simulink model "Appl_DrRestMode_CtrlModel"  (R2018b)
settings: configuration reference "CodeConfig_10_ms" (kept outside this file)
undefined symbols (not defined in the file): D_ClickNapBackPosi, D_ClickNapLengthPosi, D_DRMEM_SPEED_5, D_SoftDistanceDrLegnth, FALSE, TRUE
libraries: DareLib x81, simulink x1
(part 2 of 2)

== system Appl_DrRestMode_CtrlModel/UpDataInputInfo/InputSignalProcess2/MotorFault ==
  CC4_Flag : Inport
  MotorFault_Flag : Stateflow chart  TreatAsAtomicUnit=on
  "MotroFault_Flag " : Outport
  wires:
  MotorFault_Flag/1(MotroFault_Flag) -> "MotroFault_Flag "/1
  CC4_Flag/1 -> MotorFault_Flag/1(CC4_Flag)

== system Appl_DrRestMode_CtrlModel/UpDataInputInfo/InputSignalProcess2/OPEN ==
  CC1_Flag : Inport
  DrRes_AnyoneRelayFaultSts : Inport  Port=2
  DrRes_MassageMode_FB : Inport  Port=3
  DrRes_IVI_NapMode_SwtichSet : Inport  Port=4
  Open_Flag : Stateflow chart  TreatAsAtomicUnit=on
  "Open_Flag " : Outport
  Open_Flag_Reason : Outport  Port=2
  wires:
  DrRes_MassageMode_FB/1 -> Open_Flag/1(DrRes_MassageMode_FB)
  CC1_Flag/1 -> Open_Flag/2(CC1_Flag)
  DrRes_AnyoneRelayFaultSts/1 -> Open_Flag/4(DrRes_AnyoneRelayFaultSts)
  Open_Flag/1(Open_Flag) -> "Open_Flag "/1
  Open_Flag/2(Open_Flag_Reason) -> Open_Flag_Reason/1
  DrRes_IVI_NapMode_SwtichSet/1 -> Open_Flag/3(DrRes_IVI_NapMode_SwtichSet)

== system Appl_DrRestMode_CtrlModel/UpDataInputInfo/InputSignalProcess2/STOP ==
  DrRes_VoltMode : Inport
  CC2_Flag : Inport  Port=2
  DrRes_VoltSatisfy : Inport  Port=3
  Stop_Flag : Stateflow chart  TreatAsAtomicUnit=on
  "Stop_Flag " : Outport
  Stop_Flag_Reason : Outport  Port=2
  wires:
  Stop_Flag/2(Stop_Flag_Reason) -> Stop_Flag_Reason/1
  DrRes_VoltMode/1 -> Stop_Flag/2(DrRes_VoltMode)
  CC2_Flag/1 -> Stop_Flag/1(CC2_Flag)
  Stop_Flag/1(Stop_Flag) -> "Stop_Flag "/1
  DrRes_VoltSatisfy/1 -> Stop_Flag/3(DrRes_VoltSatisfy)

== stateflow chart Appl_DrRestMode_CtrlModel/UpDataInputInfo/InputSignalProcess1/CC3/CC3_Flag ==
  state Init
    en:
    CC3_Flag = FALSE;
  state TRUE
    en:
    CC3_Flag = TRUE;
    CC3_Reason = FALSE;
  state FALSE
    en:
    CC3_Flag = FALSE;
  Init -> TRUE [order 4] : /* !PC2 ||!PC8 ||（!PC9 && !PC10 ）
      | 诊断F101中配置字：“座椅按摩功能”！= 0x01:Ture
      | ||系统电源不处于ON档
      | ||（收到发动机为ECMD_EngineStatus！=0x2=engine running；（仅当DID F1FA中配置字：“P20PHEV_100km & P20PHEV_50km”=0x00：False时适用）
      | && 收到整车运行状态为VCU_VehRunSta！= 0x1:HV ON /0x2:Ready；（仅当DID F1FA中配置字：“P20PHEV_100km / P20PHEV_50km”=0x01：Ture时适用）） */
      | [DrRes_SeatMassageCfg != TRUE...
      | || DrRes_PowerMode != enPowerModeSts.EN_ON ...
      | || (DrRes_EngineRunFlag == TRUE || DrRes_VehicleRunFlag == TRUE) ]
  (default) -> Init
  FALSE -> TRUE : /* !PC2 ||!PC8 ||（!PC9 && !PC10 ）
      | 诊断F101中配置字：“座椅按摩功能”！= 0x01:Ture
      | ||系统电源不处于ON档
      | ||（收到发动机为ECMD_EngineStatus！=0x2=engine running；（仅当DID F1FA中配置字：“P20PHEV_100km & P20PHEV_50km”=0x00：False时适用）
      | && 收到整车运行状态为VCU_VehRunSta！= 0x1:HV ON /0x2:Ready；（仅当DID F1FA中配置字：“P20PHEV_100km / P20PHEV_50km”=0x01：Ture时适用）） */
      | [DrRes_SeatMassageCfg != TRUE...
      | || DrRes_PowerMode != enPowerModeSts.EN_ON ...
      | || (DrRes_EngineRunFlag != TRUE && DrRes_VehicleRunFlag != TRUE) ]
  Init -> FALSE [order 1] : /*CC3未置位原因 ：DrRes_SeatMassageCfg 不满足条件 */
      | [DrRes_SeatMassageCfg == TRUE]
      | {CC3_Reason = 1}
  TRUE -> FALSE [order 1] : /*CC3未置位原因 ：DrRes_SeatMassageCfg 不满足条件 */
      | [DrRes_SeatMassageCfg == TRUE]
      | {CC3_Reason = 1}
  Init -> FALSE [order 2] : /*CC3未置位原因 ：DrRes_PowerMode 不满足条件*/
      | [DrRes_PowerMode == enPowerModeSts.EN_ON]
      | {CC3_Reason = 2}
  TRUE -> FALSE [order 2] : /*CC3未置位原因 ：DrRes_PowerMode 不满足条件*/
      | [DrRes_PowerMode == enPowerModeSts.EN_ON]
      | {CC3_Reason = 2}
  Init -> FALSE [order 3] : /*CC3未置位原因 ：DrRes_EngineRunFlag/DrRes_VehicleRunFlag不满足条件 */
      | [DrRes_EngineRunFlag == TRUE && DrRes_VehicleRunFlag == TRUE]
      | {CC3_Reason = 3}
  TRUE -> FALSE [order 3] : /*CC3未置位原因 ：DrRes_EngineRunFlag/DrRes_VehicleRunFlag不满足条件 */
      | [DrRes_EngineRunFlag == TRUE || DrRes_VehicleRunFlag == TRUE]
      | {CC3_Reason = 3}
  data: TRUE parameter; FALSE parameter; DrRes_PowerMode input; DrRes_VehicleRunFlag input; DrRes_SeatMassageCfg input; DrRes_EngineRunFlag input; CC3_Flag output uint8; D_DRMEM_SPEED_5 parameter; CC3_Reason output uint8

== stateflow chart Appl_DrRestMode_CtrlModel/UpDataInputInfo/InputSignalProcess1/CallRet/GetCallRet ==
  state Ret
    state Fail
      en:
      CallRet = enResCallRet.EN_Fail;
    state Succeed
      en:
      CallRet = enResCallRet.EN_Success;
  state Init
    en:
    CallRet = enResCallRet.EN_Init;
  (default) -> Init
  Init -> Fail [order 1] : /*
      | 高度自动运行成功标志位 == FALSE
      | || 纵向自动运行成功标志位 == FALSE
      | || 靠背自动运行成功标志位 == FALSE
      | || 前部自动运行成功标志位 == FALSE
      | */
      | [DrRes_HeightAutoRunFlag == enSeatAutoRunSts.EN_SEAT_FAIL ...
      | || DrRes_LengthAutoRunFlag == enSeatAutoRunSts.EN_SEAT_FAIL ...
      | || DrRes_BackAutoRunFlag == enSeatAutoRunSts.EN_SEAT_FAIL ...
      | || DrRes_FrontAutoRunFlag == enSeatAutoRunSts.EN_SEAT_FAIL ...
      | || (DrRes_CurrentMoveType != enSeatMotorRunType.EN_ResEnable ...
      | && DrRes_CurrentMoveType != enSeatMotorRunType.EN_HUMEnable ...
      | && DrRes_CurrentMoveType != enSeatMotorRunType.EN_ComfortEnable ...
      | && DrRes_CurrentMoveType != enSeatMotorRunType.EN_MemoryEnable ...
      | && DrRes_CurrentMoveType != enSeatMotorRunType.EN_NULL)]
  Init -> Succeed [order 2] : /*(高度自动运行成功标志位 == 2 || 高度堵转)
      | && (纵向自动运行成功标志位 == 2 || 纵向堵转)
      | && (靠背自动运行成功标志位 == 2 || 靠背堵转)
      | && (前部自动运行成功标志位 == 2 || 前部堵转)*/
      | [(DrRes_HeightAutoRunFlag == enSeatAutoRunSts.EN_SEAT_SUCCESS ...
      | || DrRes_HeightLockFault == TRUE) ...
      | && (DrRes_LengthAutoRunFlag == enSeatAutoRunSts.EN_SEAT_SUCCESS ...
      |     || DrRes_LengthLockFault == TRUE) ...
      | && (DrRes_BackAutoRunFlag == enSeatAutoRunSts.EN_SEAT_SUCCESS ...
      |     || DrRes_BackLockFault == TRUE) ...
      | && (DrRes_FrontAutoRunFlag == enSeatAutoRunSts.EN_SEAT_SUCCESS ...
      |     || DrRes_FrontLockFault == TRUE)]
  Ret -> Init : [(DrRes_HeightAutoRunFlag == enSeatAutoRunSts.EN_SEAT_INVALID ...
      | && DrRes_LengthAutoRunFlag == enSeatAutoRunSts.EN_SEAT_INVALID ...
      | && DrRes_BackAutoRunFlag == enSeatAutoRunSts.EN_SEAT_INVALID ...
      | && DrRes_FrontAutoRunFlag == enSeatAutoRunSts.EN_SEAT_INVALID ...
      | && DrRes_CurrentMoveType == enSeatMotorRunType.EN_NULL) ...
      | || hasChangedTo(DrRes_CurrentMoveType,enSeatMotorRunType.EN_ResEnable)]
      | {CallRet = 0;}
  data: TRUE parameter; FALSE parameter; CallRet output uint8; DrRes_HeightAutoRunFlag input; DrRes_LengthAutoRunFlag input; DrRes_BackAutoRunFlag input; DrRes_FrontAutoRunFlag input; DrRes_HeightLockFault input; DrRes_LengthLockFault input; DrRes_BackLockFault input; DrRes_FrontLockFault input; DrRes_CurrentMoveType input

== stateflow chart Appl_DrRestMode_CtrlModel/UpDataInputInfo/InputSignalProcess2/STOP/Stop_Flag ==
  state FALSE
    en:
    Stop_Flag = FALSE;
  state Init
    en:
    Stop_Flag = FALSE;
  state TRUE
    en:
    Stop_Flag = TRUE;
    Stop_Flag_Reason = FALSE;
  Init -> TRUE [order 3] : /*!PC1||CC2
      | 电压不处于正常模式
      | ||CC2标志位 == 1*/
      | [DrRes_VoltMode != enFinalPowerMode.EN_NORMAL_VOLT  ...
      | || TRUE != DrRes_VoltSatisfy ...
      | || CC2_Flag == TRUE]
  (default) -> Init
  FALSE -> TRUE : /*!PC1||CC2
      | 电压不处于正常模式
      | ||CC2标志位 == 1*/
      | [DrRes_VoltMode != enFinalPowerMode.EN_NORMAL_VOLT  ...
      | || TRUE != DrRes_VoltSatisfy ...
      | || CC2_Flag == TRUE]
  TRUE -> FALSE [order 1] : /*Stop_Flag未置位原因 ：DrRes_VoltMode 不满足条件 */
      | [DrRes_VoltMode == enFinalPowerMode.EN_NORMAL_VOLT ...
      | && TRUE == DrRes_VoltSatisfy]
      | {Stop_Flag_Reason = 1}
  Init -> FALSE [order 1] : /*Stop_Flag未置位原因 ：DrRes_VoltMode 不满足条件 */
      | [DrRes_VoltMode == enFinalPowerMode.EN_NORMAL_VOLT ...
      | && TRUE == DrRes_VoltSatisfy]
      | {Stop_Flag_Reason = 1}
  TRUE -> FALSE [order 2] : /*Stop_Flag未置位原因 ：CC2_Flag 不满足条件 */
      | [CC2_Flag != TRUE]
      | {Stop_Flag_Reason = 2}
  Init -> FALSE [order 2] : /*Stop_Flag未置位原因 ：CC2_Flag 不满足条件 */
      | [CC2_Flag != TRUE]
      | {Stop_Flag_Reason = 2}
  data: TRUE parameter; FALSE parameter; CC2_Flag input; DrRes_VoltMode input; Stop_Flag output uint8; D_DRMEM_SPEED_5 parameter; Stop_Flag_Reason output uint8; DrRes_VoltSatisfy input

== stateflow chart Appl_DrRestMode_CtrlModel/UpDataInputInfo/InputSignalProcess1/GetHallValue/Char_CallHallVall_Length ==
  state Char_CallHallVall_Length
    en:Temp_Drs_Distance = (DrRes_LengthDefaultMotorSize * D_ClickNapLengthPosi)/100;
    du:
    Char_CallHallVall_Length -> (junction 187)
    (junction 187) -> (junction 194) : /*计算后移坐标与后软止点坐标  */
        | {Temp_Drs_Posi = DrRes_LengthHallPosi -  Temp_Drs_Distance;
        | Temp_Drs_SoftStopPosi = (DrRes_LengthDefaultStopPos + D_SoftDistanceDrLegnth)}
    (junction 194) -> (junction 205) [order 1] : /*后移坐标大于软止点坐标 - 可移动到后移坐标 */
        | [Temp_Drs_Posi > Temp_Drs_SoftStopPosi]
    (junction 194) -> (junction 186) [order 2]
    (junction 205) -> (junction 191) : {CallHallVall_Length = Temp_Drs_Posi}
    (junction 186) -> (junction 185) [order 1] : /* 当前坐标小于后止点坐标 不动作*/
        | [DrRes_LengthHallPosi <= Temp_Drs_SoftStopPosi]
    (junction 186) -> (junction 198) [order 2] : {CallHallVall_Length = Temp_Drs_SoftStopPosi}
    (junction 185) -> (junction 189) : {CallHallVall_Length = 0;}
    (junction 189) -> (junction 198)
    (junction 191) -> (junction 189)
    (junction 198) -> (junction 200)
  data: DrRes_LengthDefaultStopPos input; DrRes_LengthDefaultMotorSize input; DrRes_LengthHallPosi input; D_ClickNapLengthPosi input; D_SoftDistanceDrLegnth input; CallHallVall_Length output uint16; Temp_Drs_SoftStopPosi local uint32; Temp_Drs_Posi local uint32; Temp_Drs_Distance local uint32

== stateflow chart Appl_DrRestMode_CtrlModel/UpDataInputInfo/InputSignalProcess1/CC2/CC2_Flag ==
  state Init
    en:
    CC2_Flag = FALSE;
  state FALSE
    en:
    CC2_Flag = FALSE;
  state TRUE
    en:
    CC2_Flag = TRUE;
    CC2_Reason = FALSE;
  Init -> TRUE [order 4] : /* !PC3 ||!PC4 ||!PC5
      | 诊断F101中配置字：“主驾座椅调节”！= 0x02:Twelve way motor
      | || 诊断F101中配置字：“主驾记忆迎宾功能”！=0x01: TRUE
      | ||主驾座椅未学习 */
      | [DrRes_AdjustEnable != enAdjustEnable.EN_TwelveWayMotor ...
      | || DrRes_WelcomeEnable != TRUE ...
      | || DrRes_SeatLearnResult != TRUE]
  (default) -> Init
  FALSE -> TRUE : /* !PC3 ||!PC4 ||!PC5
      | 诊断F101中配置字：“主驾座椅调节”！= 0x02:Twelve way motor
      | || 诊断F101中配置字：“主驾记忆迎宾功能”！=0x01: TRUE
      | ||主驾座椅未学习 */
      | [DrRes_AdjustEnable != enAdjustEnable.EN_TwelveWayMotor ...
      | || DrRes_WelcomeEnable != TRUE ...
      | || DrRes_SeatLearnResult != TRUE]
  Init -> FALSE [order 1] : /*CC2未置位原因 ：DrRes_AdjustEnable不满足条件 */
      | [DrRes_AdjustEnable == enAdjustEnable.EN_TwelveWayMotor]
      | {CC2_Reason = 1}
  TRUE -> FALSE [order 1] : /*CC2未置位原因 ：DrRes_AdjustEnable不满足条件 */
      | [DrRes_AdjustEnable == enAdjustEnable.EN_TwelveWayMotor]
      | {CC2_Reason = 1}
  Init -> FALSE [order 2] : /*CC2未置位原因 ：DrRes_WelcomeEnable 不满足条件*/
      | [DrRes_WelcomeEnable == TRUE]
      | {CC2_Reason = 2}
  TRUE -> FALSE [order 2] : /*CC2未置位原因 ：DrRes_WelcomeEnable 不满足条件*/
      | [DrRes_WelcomeEnable == TRUE]
      | {CC2_Reason = 2}
  Init -> FALSE [order 3] : /*CC2未置位原因 ：DrRes_SeatLearnResult不满足条件 */
      | [DrRes_SeatLearnResult == TRUE]
      | {CC2_Reason = 3}
  TRUE -> FALSE [order 3] : /*CC2未置位原因 ：DrRes_SeatLearnResult不满足条件 */
      | [DrRes_SeatLearnResult == TRUE]
      | {CC2_Reason = 3}
  data: TRUE parameter; FALSE parameter; DrRes_SeatLearnResult input; DrRes_AdjustEnable input; DrRes_WelcomeEnable input; CC2_Flag output uint8; D_DRMEM_SPEED_5 parameter; CC2_Reason output uint8

== stateflow chart Appl_DrRestMode_CtrlModel/UpDataInputInfo/InputSignalProcess1/CC4/CC4_Flag ==
  state FALSE
    en:
    CC4_Flag = FALSE;
  state TRUE
    en:
    CC4_Flag = TRUE;
    CC4_Reason = FALSE;
  (default) -> FALSE
  FALSE -> TRUE : /* C6 & C7
      | 无主驾座椅任一方向霍尔故障 */
      | [DrRes_DescHeightHallFault != TRUE ...
      | && DrRes_DescLengthHallFault  != TRUE ...
      | && DrRes_DescBackHallFault  != TRUE ...
      | && DrRes_DescFrontHallFault  != TRUE ...
      | && DrRes_HeightLockFault  != TRUE ...
      | && DrRes_LengthLockFault  != TRUE ...
      | && DrRes_BackLockFault  != TRUE ...
      | && DrRes_FrontLockFault  != TRUE]
  TRUE -> FALSE : /*CC4未置位原因 ：DrRes_AnyoneHallFaultSts 不满足条件*/
      | [DrRes_DescHeightHallFault == TRUE ...
      | || DrRes_DescLengthHallFault  == TRUE ...
      | || DrRes_DescBackHallFault  == TRUE ...
      | || DrRes_DescFrontHallFault  == TRUE ...
      | || DrRes_HeightLockFault == TRUE ...
      | || DrRes_LengthLockFault  == TRUE ...
      | || DrRes_BackLockFault  == TRUE ...
      | || DrRes_FrontLockFault  == TRUE]
      | {CC4_Reason = 1}
  data: TRUE parameter; FALSE parameter; DrRes_DescHeightHallFault input; CC4_Flag output uint8; CC4_Reason output uint8; DrRes_DescBackHallFault input; DrRes_DescFrontHallFault input; DrRes_DescLengthHallFault input; DrRes_LengthLockFault input; DrRes_BackLockFault input; DrRes_FrontLockFault input; DrRes_HeightLockFault input

== stateflow chart Appl_DrRestMode_CtrlModel/LogicCtrl/ResCtrl/ResDeal ==
  state SaveResReCallPosi(In1,ln2,In3,ln4) [function]
  state SetResCallPosi(In1,ln2,In3,ln4) [function]
  state Inactive
    en:
    DSM_NapMode_FB = enNapMode.EN_NapMode_Close;
    state WaitInit
      en:
      SaveReTimer = 0;
      WaitTimer = 0;
      StartFlag = 0;
      du:
      WaitTimer += 1;
      ex:
      SaveReTimer = 3;
    state Init
      en:
      ResCallPosi_Height = 0;
      ResCallPosi_Length = 0;
      ResCallPosi_Back = 0;
      ResCallPosi_Front = 0;
      State_ResDeal = 1;
      StartFlag = TRUE;
      SavePosiCnt = 10;
      ex:
      SaveReTimer = 0;
      (default) -> (junction 187)
      Init -> (junction 187)
      (junction 187) -> (junction 238) [order 1] : /* 延迟20ms存储 */
          | [SaveReTimer  > 2]
      (junction 238) -> (junction 240) [order 1] : [hasChangedTo(DrRes_CurrentMoveType,0) ...
          | || DrResl_ReCallPosi_Height == 0 ...
          | || DrResl_ReCallPosi_Length == 0 ...
          | || DrResl_ReCallPosi_Back == 0 ...
          | || DrResl_ReCallPosi_Front == 0 ...
          | || DrResl_ReCallPosi_Height == 0xFFFF ...
          | || DrResl_ReCallPosi_Length == 0xFFFF ...
          | || DrResl_ReCallPosi_Back == 0xFFFF ...
          | || DrResl_ReCallPosi_Front == 0xFFFF]
      (junction 187) -> (junction 247) [order 2] : {SaveReTimer ++;}
      (junction 238) -> (junction 244) [order 2]
      (junction 240) -> (junction 242) : {SavePosiCnt = 0;}
      (junction 244) -> (junction 247)
      (junction 242) -> (junction 244)
      (junction 247) -> (junction 268)
      (junction 268) -> (junction 270) [order 1] : /* 缓存次数未超 */
          | [SavePosiCnt < 10]
      (junction 268) -> (junction 274) [order 2]
      (junction 270) -> (junction 272) : /* 更新回位位置 */
          | {SaveResReCallPosi ...
          | (DrRes_HeightHallPosi, ...
          | DrRes_LengthHallPosi, ...
          | DrRes_BackHallPosi, ...
          | DrRes_FrontHallPosi);
          | SavePosiCnt++;}
      (junction 272) -> (junction 274)
      (junction 274) -> (junction 250) : {TempCallPosi_Height = CallHallVall_Height;
          | TempCallPosi_Length = CallHallVall_Length;
          | TempCallPosi_Back = CallHallVall_Back;
          | TempCallPosi_Front = CallHallVall_Front;
          | SetResCallPosi(TempCallPosi_Height, TempCallPosi_Length,...
          |  TempCallPosi_Back, TempCallPosi_Front)}
    state ReCall
      en:
      State_ResDeal = 2;
    (default) -> WaitInit
    WaitInit -> Init : /* 位置读取完成 */
        | [WaitTimer >= 20]
    ReCall -> Init [order 2] : /*小憩调用成功标志==1
        | ||小憩调用失败标志==1
        | ||小憩停止动作标志==1*/
        | [Stop_Flag == TRUE ...
        | || DrRestCAll_Ret != enResCallRet.EN_Init]
  state Active
    en:
    DSM_NapMode_FB = enNapMode.EN_NapMode_Open;
    note: 调用位置=标定坐标 纵向距前硬止点80mm、靠背距前硬止点65°、高度和前部保持不动
    state Call
      en:
      State_ResDeal = 3;
      ResCallPosi_Height = TempCallPosi_Height;
      ResCallPosi_Length = TempCallPosi_Length;
      ResCallPosi_Back = TempCallPosi_Back;
      ResCallPosi_Front = TempCallPosi_Front;
      DSM_MassageLevel_Req=enMassageLevel_DSM.EN_L3;
      DSM_MassageMode_Req=enMassageMode_DSM.EN_M1
      RestReUpdatePosiFlag = 0;
    state CallOver
      en:
      State_ResDeal = 4;
      ResCallPosi_Height = 0;
      ResCallPosi_Length = 0;
      ResCallPosi_Back = 0;
      ResCallPosi_Front = 0;
    Call -> CallOver [order 2] : /*小憩调用成功标志==1
        | ||小憩调用失败标志==1*/
        | [DrRestCAll_Ret != enResCallRet.EN_Init]
  state Fault
    en:
    State_ResDeal = 5;
    DSM_NapMode_FB = EN_NapMode_ERR;
    ResCallPosi_Height = 0;
    ResCallPosi_Length = 0;
    ResCallPosi_Back = 0;
    ResCallPosi_Front = 0;
    RestReUpdatePosiFlag = 1;
  (default) -> Inactive
  Inactive -> Call [commented out] : /*小憩开启请求标志==1 && 需要更新回位位置
      | /回位位置=当前坐标*/
      | [Open_Flag == TRUE && RestReUpdatePosiFlag == 1]
      | {SaveResReCallPosi(DrRes_HeightHallPosi, ...
      | DrRes_LengthHallPosi, DrRes_BackHallPosi, DrRes_FrontHallPosi);
      | ResReCallPosi_Height = DrRes_HeightHallPosi;
      | ResReCallPosi_Length = DrRes_LengthHallPosi;
      | ResReCallPosi_Back = DrRes_BackHallPosi;
      | ResReCallPosi_Front = DrRes_FrontHallPosi;}
  Inactive -> Call [order 2] : /*小憩开启请求标志==1 且时间已等待完毕
      | /回位位置=上一次的回位坐标*/
      | [Open_Flag == TRUE && WaitTimer >= 20 ...
      | && StartFlag == TRUE]
      | {ResReCallPosi_Height = DrResl_ReCallPosi_Height;
      | ResReCallPosi_Length = DrResl_ReCallPosi_Length;
      | ResReCallPosi_Back = DrResl_ReCallPosi_Back;
      | ResReCallPosi_Front = DrResl_ReCallPosi_Front;}
  Active -> Init [order 3] : /*小憩停止动作标志==1*/
      | [Stop_Flag == TRUE]
      | {DSM_MassageLevel_Req=enMassageLevel_DSM.EN_OFF;}
  Call -> Fault [order 1] : /*电机故障标志位==1*/
      | [MotorFault_Flag == 1]
      | {DSM_MassageLevel_Req=enMassageLevel_DSM.EN_OFF;}
  Fault -> Init : /*按摩故障标志位==0
      | && 电机故障标志位==0
      | && 继电器粘连故障状态==0*/
      | [(MassageFault_Flag == 0 ...
      | && MotorFault_Flag == 0 ...
      | && DrRes_AnyoneRelayFaultSts == 0)]
  Active -> ReCall [order 2] : /*小憩关闭请求标志==1*/
      | [Close_Flag == TRUE]
      | {ResCallPosi_Height = DrResl_ReCallPosi_Height;
      | ResCallPosi_Length = DrResl_ReCallPosi_Length;
      | ResCallPosi_Back = DrResl_ReCallPosi_Back;
      | ResCallPosi_Front = DrResl_ReCallPosi_Front;
      | DSM_MassageLevel_Req=enMassageLevel_DSM.EN_OFF;}
  ReCall -> Fault [order 1] : /*电机故障标志位==1
      | ||按摩故障标志位==1
      | ||继电器粘连故障状态==1*/
      | [MotorFault_Flag == 1 ...
      | ||MassageFault_Flag == 1 ...
      | || DrRes_AnyoneRelayFaultSts == 1]
      | {DSM_MassageLevel_Req=enMassageLevel_DSM.EN_OFF;}
  Active -> Fault [order 1] : /*
      | ||按摩故障标志位==1*/
      | [MassageFault_Flag == 1 ...
      | || DrRes_AnyoneRelayFaultSts == 1]
      | {DSM_MassageLevel_Req=enMassageLevel_DSM.EN_OFF;}
  Inactive -> Fault [order 1] : /*小憩开启请求标志==1
      | && (按摩故障标志位==1
      | || 继电器粘连故障状态==1*/
      | [Open_Flag == TRUE ...
      | && (MassageFault_Flag == 1 ...
      | || DrRes_AnyoneRelayFaultSts == 1)]
      | {DSM_MassageLevel_Req=enMassageLevel_DSM.EN_OFF;}
  data: In1 function_input; ln2 function_input; In3 function_input; ln4 function_input; In1 function_input; ln2 function_input; In3 function_input; ln4 function_input; DSM_MassageLevel_Req output uint8; DSM_MassageMode_Req output uint8; DSM_NapMode_FB output uint8; FALSE parameter; DrResl_ReCallPosi_Height input; DrResl_ReCallPosi_Length input; DrResl_ReCallPosi_Back input; DrResl_ReCallPosi_Front input; CallHallVall_Height input; CallHallVall_Length input; CallHallVall_Back input; CallHallVall_Front input; DrRes_HeightHallPosi input; TRUE parameter; DrRes_LengthHallPosi input; DrRes_BackHallPosi input; DrRes_FrontHallPosi input; Stop_Flag input; Open_Flag input; Close_Flag input; ResCallPosi_Height output uint16; ResCallPosi_Length output uint16; ResCallPosi_Front output uint16; ResCallPosi_Back output uint16; ResReCallPosi_Back output uint16; ResReCallPosi_Front output uint16; ResReCallPosi_Height output uint16; ResReCallPosi_Length output uint16; MotorFault_Flag input; State_ResDeal output uint8; RestReUpdatePosiFlag local uint8; WaitTimer local uint8; MassageFault_Flag input; DrRes_AnyoneRelayFaultSts input; DrRestCAll_Ret input; SaveReTimer local uint8; TempCallPosi_Height local uint16; TempCallPosi_Length local uint16; TempCallPosi_Back local uint16; TempCallPosi_Front local uint16; DrRes_CurrentMoveType input; StartFlag local uint8; SavePosiCnt local uint8; StartFlag1 local uint8

== stateflow chart Appl_DrRestMode_CtrlModel/UpDataInputInfo/InputSignalProcess1/CC1/CC1_Flag ==
  state Init
    en:
    CC1_Flag = TRUE;
    CC1_Reason = FALSE;
  state FALSE
    en:
    CC1_Flag = FALSE;
  state TRUE
    en:
    CC1_Flag = TRUE;
    CC1_Reason = FALSE;
  Init -> TRUE [order 9] : /*PC1&&PC2&&PC3&&PC4 &&PC5&&PC6&&PC8
      | &&(PC9 ||PC10)
      |
      | 电压处于正常模式
      | &&诊断F101中配置字：“座椅按摩功能”= 0x01:Ture
      | &&诊断F101中配置字：“主驾座椅调节”= 0x02:Twelve way motor
      | &&诊断F101中配置字：“主驾记忆迎宾功能”=0x01: TRUE
      | &&主驾座椅已学习
      | &&主驾座椅各方向电机均不处于本地调节运动中
      | &&系统电源处于ON档
      | &&（收到发动机为ECMD_EngineStatus=0x2=engine running；（仅当DID F1FA中配置字：“P20PHEV_100km & P20PHEV_50km”=0x00：False时适用）
      | || 收到整车运行状态为VCU_VehRunSta= 0x1:HV ON /0x2:Ready；（仅当DID F1FA中配置字：“P20PHEV_100km / P20PHEV_50km”=0x01：Ture时适用））*/
      | [DrRes_VoltMode == enFinalPowerMode.EN_NORMAL_VOLT ...
      | && TRUE == DrRes_VoltSatisfy ...
      | && DrRes_SeatMassageCfg == TRUE...
      | &&  DrRes_AdjustEnable == enAdjustEnable.EN_TwelveWayMotor ...
      | && DrRes_WelcomeEnable == TRUE ...
      | && DrRes_SeatLearnResult == TRUE ...
      | && DrRes_CurrentMoveType != enSeatMotorRunType.EN_ManualEnable ...
      | && DrRes_PowerMode == enPowerModeSts.EN_ON ...
      | && (DrRes_EngineRunFlag == TRUE || DrRes_VehicleRunFlag == TRUE)]
  (default) -> Init
  FALSE -> TRUE : /*PC1&&PC2&&PC3&&PC4 &&PC5&&PC6&&PC8
      | &&(PC9 ||PC10)
      |
      | 电压处于正常模式
      | &&诊断F101中配置字：“座椅按摩功能”= 0x01:Ture
      | &&诊断F101中配置字：“主驾座椅调节”= 0x02:Twelve way motor
      | &&诊断F101中配置字：“主驾记忆迎宾功能”=0x01: TRUE
      | &&主驾座椅已学习
      | &&主驾座椅各方向电机均不处于本地调节运动中
      | &&系统电源处于ON档
      | &&（收到发动机为ECMD_EngineStatus=0x2=engine running；（仅当DID F1FA中配置字：“P20PHEV_100km & P20PHEV_50km”=0x00：False时适用）
      | || 收到整车运行状态为VCU_VehRunSta= 0x1:HV ON /0x2:Ready；（仅当DID F1FA中配置字：“P20PHEV_100km / P20PHEV_50km”=0x01：Ture时适用））*/
      | [DrRes_VoltMode == enFinalPowerMode.EN_NORMAL_VOLT ...
      | && TRUE == DrRes_VoltSatisfy ...
      | && DrRes_SeatMassageCfg == TRUE...
      | &&  DrRes_AdjustEnable == enAdjustEnable.EN_TwelveWayMotor ...
      | && DrRes_WelcomeEnable == TRUE ...
      | && DrRes_SeatLearnResult == TRUE ...
      | && DrRes_CurrentMoveType != enSeatMotorRunType.EN_ManualEnable ...
      | && DrRes_PowerMode == enPowerModeSts.EN_ON ...
      | && (DrRes_EngineRunFlag == TRUE || DrRes_VehicleRunFlag == TRUE)]
  Init -> FALSE [order 1] : /*CC1未置位原因 ：DrRes_VoltMode不满足条件 */
      | [DrRes_VoltMode != enFinalPowerMode.EN_NORMAL_VOLT ...
      | || TRUE != DrRes_VoltSatisfy]
      | {CC1_Reason = 1}
  TRUE -> FALSE [order 1] : /*CC1未置位原因 ：DrRes_VoltMode不满足条件 */
      | [DrRes_VoltMode != enFinalPowerMode.EN_NORMAL_VOLT ...
      | || TRUE != DrRes_VoltSatisfy]
      | {CC1_Reason = 1}
  Init -> FALSE [order 2] : /*CC1未置位原因 ：DrRes_SeatMassageCfg不满足条件 */
      | [DrRes_SeatMassageCfg != TRUE]
      | {CC1_Reason = 2}
  TRUE -> FALSE [order 2] : /*CC1未置位原因 ：DrRes_SeatMassageCfg不满足条件 */
      | [DrRes_SeatMassageCfg != TRUE]
      | {CC1_Reason = 2}
  Init -> FALSE [order 3] : /*CC1未置位原因 ：DrRes_AdjustEnable 不满足条件*/
      | [DrRes_AdjustEnable != enAdjustEnable.EN_TwelveWayMotor]
      | {CC1_Reason = 3}
  TRUE -> FALSE [order 3] : /*CC1未置位原因 ：DrRes_AdjustEnable 不满足条件*/
      | [DrRes_AdjustEnable != enAdjustEnable.EN_TwelveWayMotor]
      | {CC1_Reason = 3}
  TRUE -> FALSE [order 4] : /*CC1未置位原因 ：DrRes_WelcomeEnable不满足条件 */
      | [DrRes_WelcomeEnable != TRUE]
      | {CC1_Reason = 4}
  Init -> FALSE [order 4] : /*CC1未置位原因 ：DrRes_WelcomeEnable不满足条件 */
      | [DrRes_WelcomeEnable != TRUE]
      | {CC1_Reason = 4}
  TRUE -> FALSE [order 5] : /*CC1未置位原因 ：DrRes_SeatLearnResult 不满足条件*/
      | [DrRes_SeatLearnResult != TRUE]
      | {CC1_Reason = 5}
  Init -> FALSE [order 5] : /*CC1未置位原因 ：DrRes_SeatLearnResult 不满足条件*/
      | [DrRes_SeatLearnResult != TRUE]
      | {CC1_Reason = 5}
  Init -> FALSE [order 6] : /*CC1未置位原因 ：DrRes_CurrentMoveType不满足条件 */
      | [DrRes_CurrentMoveType == enSeatMotorRunType.EN_ManualEnable]
      | {CC1_Reason = 6}
  TRUE -> FALSE [order 6] : /*CC1未置位原因 ：DrRes_CurrentMoveType不满足条件 */
      | [DrRes_CurrentMoveType == enSeatMotorRunType.EN_ManualEnable]
      | {CC1_Reason = 6}
  Init -> FALSE [order 7] : /*CC1未置位原因 ：DrRes_PowerMode不满足条件 */
      | [DrRes_PowerMode != enPowerModeSts.EN_ON]
      | {CC1_Reason = 7}
  TRUE -> FALSE [order 7] : /*CC1未置位原因 ：DrRes_PowerMode不满足条件 */
      | [DrRes_PowerMode != enPowerModeSts.EN_ON]
      | {CC1_Reason = 7}
  Init -> FALSE [order 8] : /*CC1未置位原因 ：DrRes_EngineRunFlag/：DrRes_VehicleRunFlag不满足条件 */
      | [DrRes_EngineRunFlag != TRUE && DrRes_VehicleRunFlag != TRUE ]
      | {CC1_Reason = 8}
  TRUE -> FALSE [order 8] : /*CC1未置位原因 ：DrRes_EngineRunFlag/：DrRes_VehicleRunFlag不满足条件 */
      | [DrRes_EngineRunFlag != TRUE && DrRes_VehicleRunFlag != TRUE ]
      | {CC1_Reason = 8}
  data: TRUE parameter; FALSE parameter; DrRes_EngineRunFlag input; DrRes_PowerMode input; DrRes_CurrentMoveType input; DrRes_WelcomeEnable input; DrRes_SeatLearnResult input; DrRes_AdjustEnable input; DrRes_VehicleRunFlag input; DrRes_VoltMode input; DrRes_SeatMassageCfg input; CC1_Flag output uint8; D_DRMEM_SPEED_5 parameter; CC1_Reason output uint8; DrRes_VoltSatisfy input

== stateflow chart Appl_DrRestMode_CtrlModel/UpDataInputInfo/InputSignalProcess2/OPEN/Open_Flag ==
  state FALSE
    en:
    Open_Flag = FALSE;
  state Ready
    en:
    Open_Flag = FALSE;
    Open_Flag_Reason = FALSE;
    RequestTimer = 0;
  state Open
    en:
    Open_Flag = TRUE;
    Open_Flag_Reason = FALSE;
    RequestTimer = 0;
    du:
    RequestTimer ++;
  state Init
    en:
    Open_Flag = FALSE;
  Init -> Ready [order 2] : /* CC1&&PC7&&PC11&&C4
      | CC1标志位 == 1
      | && 无主驾座椅任一方向继电器粘连故障
      | && 按摩模块无故障：DSM_MassageMode_FB≠0x8：Error模块故障
      | */
      | [CC1_Flag == TRUE ]
  (default) -> Init
  FALSE -> Ready : /* CC1&&PC7&&PC11&&C4
      | CC1标志位 == 1
      | && 无主驾座椅任一方向继电器粘连故障
      | && 按摩模块无故障：DSM_MassageMode_FB≠0x8：Error模块故障
      | */
      | [CC1_Flag == TRUE]
  Ready -> Open [order 2] : /* CC1&&PC7&&PC11&&C4
      | 收到小憩模式请求信号（IVI_NapMode_SwtichSet）＝0x1:打开小憩模式 */
      | [DrRes_IVI_NapMode_SwtichSet == 1]
  Ready -> FALSE [order 1] : /*Open_Flag未置位原因 ：CC1_Flag不满足条件 */
      | [CC1_Flag != TRUE]
      | {Open_Flag_Reason = 1}
  Init -> FALSE [order 1] : /*Open_Flag未置位原因 ：CC1_Flag不满足条件 */
      | [CC1_Flag != TRUE]
      | {Open_Flag_Reason = 1}
  Ready -> FALSE [commented out] : /*Open_Flag未置位原因 ：DrRes_AnyoneRelayFaultSts不满足条件 */
      | [DrRes_AnyoneRelayFaultSts == TRUE]
      | {Open_Flag_Reason = 2}
  Init -> FALSE [commented out] : /*Open_Flag未置位原因 ：DrRes_AnyoneRelayFaultSts不满足条件 */
      | [DrRes_AnyoneRelayFaultSts == TRUE]
      | {Open_Flag_Reason = 2}
  Open -> Ready : [RequestTimer >= 20]
  Ready -> FALSE [commented out] : /*Open_Flag未置位原因 ：DrRes_MassageMode_FB不满足条件 */
      | [DrRes_MassageMode_FB == enMassageMode_DSM.EN_MError]
      | {Open_Flag_Reason = 3}
  Init -> FALSE [commented out] : /*Open_Flag未置位原因 ：DrRes_MassageMode_FB不满足条件 */
      | [DrRes_MassageMode_FB == enMassageMode_DSM.EN_MError]
      | {Open_Flag_Reason = 3}
  data: TRUE parameter; FALSE parameter; DrRes_MassageMode_FB input; CC1_Flag input; DrRes_IVI_NapMode_SwtichSet input; DrRes_AnyoneRelayFaultSts input; Open_Flag output uint8; D_DRMEM_SPEED_5 parameter; Open_Flag_Reason output uint8; RequestTimer local uint8

== stateflow chart Appl_DrRestMode_CtrlModel/UpDataInputInfo/InputSignalProcess2/CLOSE/Colse_Flag ==
  state Init
    state Init
      en:
      Close_Flag = FALSE;
    state FALSE
      en:
      Close_Flag = FALSE;
    state Ready
      en:
      Close_Flag = FALSE;
      Close_Flag_Reason = FALSE;
      RequestTimer = 0;
    Init.Init -> Ready [order 3] : /* (PC7&&PC11&&C5)||CC3
        | 无主驾座椅任一方向继电器粘连故障
        | && 按摩模块无故障：DSM_MassageMode_FB≠0x8：Error模块故障
        |  */
        | [DrRes_AnyoneRelayFaultSts != TRUE ...
        | || DrRes_MassageMode_FB != enMassageMode_DSM.EN_MError]
    (default) -> Init.Init
    FALSE -> Ready : /* (PC7&&PC11&&C5)||CC3
        | 无主驾座椅任一方向继电器粘连故障
        | && 按摩模块无故障：DSM_MassageMode_FB≠0x8：Error模块故障
        |  */
        | [DrRes_AnyoneRelayFaultSts != TRUE ...
        | || DrRes_MassageMode_FB != enMassageMode_DSM.EN_MError]
    Init.Init -> FALSE [order 1] : /*Close_Flag未置位原因 ：DrRes_AnyoneRelayFaultSts不满足条件 */
        | [DrRes_AnyoneRelayFaultSts == TRUE]
        | {Close_Flag_Reason = 1}
    Ready -> FALSE [order 1] : /*Close_Flag未置位原因 ：DrRes_AnyoneRelayFaultSts不满足条件 */
        | [DrRes_AnyoneRelayFaultSts == TRUE]
        | {Close_Flag_Reason = 1}
    Ready -> FALSE [order 2] : /*Close_Flag未置位原因 ：DrRes_MassageMode_FB不满足条件 */
        | [DrRes_MassageMode_FB == enMassageMode_DSM.EN_MError]
        | {Close_Flag_Reason = 2}
    Init.Init -> FALSE [order 2] : /*Close_Flag未置位原因 ：DrRes_MassageMode_FB不满足条件 */
        | [DrRes_MassageMode_FB == enMassageMode_DSM.EN_MError]
        | {Close_Flag_Reason = 2}
  state CLOSE
    en:
    Close_Flag = TRUE;
    RequestTimer = 0;
    du:
    RequestTimer ++;
  (default) -> Init
  Ready -> CLOSE [order 3] : /*收到小憩模式请求信号（IVI_NapMode_SwtichSet）＝0x2:关闭小憩模式*/
      | [DrRes_IVI_NapMode_SwtichSet == 2]
  Init -> CLOSE : [CC3_Flag == TRUE]
  CLOSE -> Init : [RequestTimer >= 20 ...
      | && CC3_Flag != TRUE ]
  data: TRUE parameter; FALSE parameter; DrRes_MassageMode_FB input; DrRes_IVI_NapMode_SwtichSet input; DrRes_AnyoneRelayFaultSts input; CC3_Flag input; Close_Flag output uint8; D_DRMEM_SPEED_5 parameter; Close_Flag_Reason output uint8; RequestTimer local uint8

== stateflow chart Appl_DrRestMode_CtrlModel/UpDataInputInfo/InputSignalProcess2/MotorFault/MotorFault_Flag ==
  state FALSE
    en:
    MotroFault_Flag = FALSE;
  state TRUE
    en:
    MotroFault_Flag = TRUE;
  (default) -> TRUE
  FALSE -> TRUE : /* ！CC4
      | CC4标志位 == 0 */
      | [CC4_Flag == 0]
  TRUE -> FALSE : [CC4_Flag == TRUE]
  data: TRUE parameter; FALSE parameter; CC4_Flag input; MotroFault_Flag output uint8; D_DRMEM_SPEED_5 parameter

== stateflow chart Appl_DrRestMode_CtrlModel/UpDataInputInfo/InputSignalProcess2/MassageFault/MassageFault_Flag ==
  state FALSE
    en:
    MassageFault_Flag = FALSE;
  state TRUE
    en:
    MassageFault_Flag = TRUE;
  (default) -> TRUE
  FALSE -> TRUE : /* ！PC11
      | 按摩模块无故障：DSM_MassageMode_FB==0x8：Error模块故障*/
      | [DrRes_MassageMode_FB == enMassageMode_DSM.EN_MError]
  TRUE -> FALSE : [DrRes_MassageMode_FB != enMassageMode_DSM.EN_MError]
  data: TRUE parameter; FALSE parameter; DrRes_MassageMode_FB input; MassageFault_Flag output uint8; D_DRMEM_SPEED_5 parameter
